simulink model "var_manip"  (R2014a)
settings: Solver=ode45  StartTime=0.0  StopTime=200  RelTol=1e-6
settings Model: Creator=sebar  LastModifiedBy=sebar

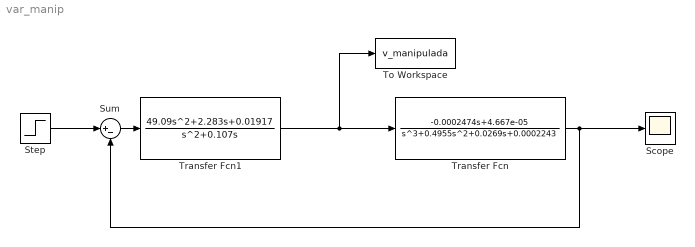
== system var_manip ==
  Scope : Scope
  Step : Step  Time=0  SampleTime=0
  Sum : Sum  Inputs=|+-
  To Workspace : ToWorkspace  VariableName=v_manipulada  SaveFormat=Structure With Time  SampleTime=-1
  Transfer Fcn : TransferFcn  Numerator=[-0.0002474 4.667e-05]  Denominator=[ 1 0.4955 0.0269 0.0002243]
  Transfer Fcn1 : TransferFcn  Numerator=[49.09 2.283 0.01917]  Denominator=[1 0.107 0]
  wires:
  Transfer Fcn/1 -> Sum/2, Scope/1
  Sum/1 -> Transfer Fcn1/1
  Transfer Fcn1/1 -> Transfer Fcn/1, To Workspace/1
  Step/1 -> Sum/1
